simulink model "ModelTests"  (R2017a)
settings: Solver=FixedStepAuto  StartTime=0.0  StopTime=10  FixedStep=0.005  RelTol=1e-3
libraries: cstblocks x3
settings Model: Creator=roman  LastModifiedBy=roman

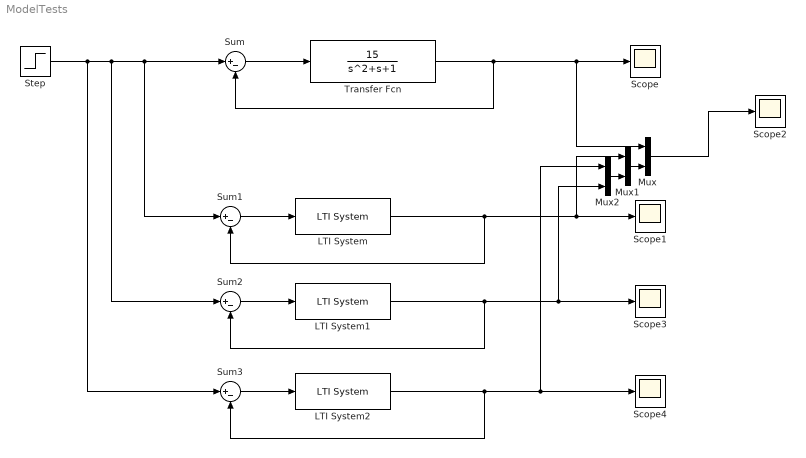
== system ModelTests ==
  LTI System : cstblocks/LTI System  sys=ss1  IC=[]
  LTI System1 : cstblocks/LTI System  sys=ss2  IC=[]
  LTI System2 : cstblocks/LTI System  sys=ss3  IC=[]
  Mux : Mux  Inputs=2
  Mux1 : Mux  Inputs=2
  Mux2 : Mux  Inputs=2
  Scope{,1..4} (5 alike) : Scope
  Step : Step  SampleTime=0
  Sum{,1..3} (4 alike) : Sum  Inputs=|+-
  Transfer Fcn : TransferFcn  Numerator=[15]  Denominator=[1 1 1]
  wires:
  Transfer Fcn/1 -> Sum/2, Scope/1, Mux/1
  Sum/1 -> Transfer Fcn/1
  Sum1/1 -> LTI System/1
  Mux/1 -> Scope2/1
  LTI System/1 -> Mux1/1, Scope1/1, Sum1/2
  LTI System1/1 -> Mux2/2, Scope3/1, Sum2/2
  Sum2/1 -> LTI System1/1
  Step/1 -> Sum3/1, Sum2/1, Sum1/1, Sum/1
  LTI System2/1 -> Scope4/1, Mux2/1, Sum3/2
  Sum3/1 -> LTI System2/1
  Mux1/1 -> Mux/2
  Mux2/1 -> Mux1/2
